simulink model "pid_test_model"  (R2018b)
settings: Solver=VariableStepAuto  StartTime=0.0  StopTime=2  RelTol=1e-3
libraries: nesl_utility x6, elec_lib x4, fl_lib x4, peGeneralControl x3, powerlib_meascontrol x2, simulink_extras x1
settings Model: Creator=macke  LastModifiedBy=macke

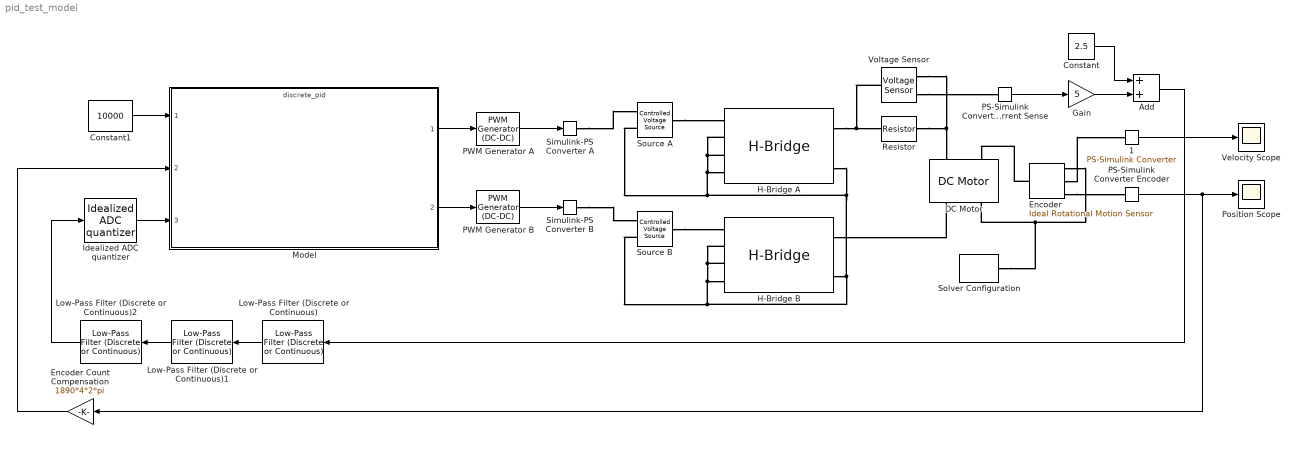
== system pid_test_model ==
  1 : nesl_utility/PS-Simulink Converter  PhysicalDomain=network_engine_domain  SubClassName=ps_output  LeftPortType=input  RightPortType=output  PseudoPeriodic=off  Frequencies=[]  Unit=1  AffineConversion=off
  Add : Sum
  Constant : Constant  Value=2.5
  Constant1 : Constant  Value=10000
  DC Motor : elec_lib/Actuators & Drivers/Rotational Actuators/DC Motor  parameterization=3  Ra=3.9 Ohm  La=12e-6 H  emf_or_torque=1  Kv=0.072e-3 V/rpm  Ki=6.876e-4 N*m/A  T_stall=0.24e-3 N*m  w_max=16.7 rpm  w_rated=12 rpm  P_rated=1.722 W  V_rated=12 V  J=0.01 g*cm^2  lam_param=2  lam=0 N*m/(rad/s)  i_noload=0.1 A  V_i_noload=12 V  speed0=0 rpm  alpha=3.93e-3 1/K  Tmeas=25 degC  thermal_mass=100 J/K  initial_temperature=25 degC
  Encoder : fl_lib/Mechanical/Mechanical Sensors/Ideal Rotational Motion Sensor  offset=0 rad
  Encoder Count Compensation : Gain  Gain=1890*4*2*pi
  Gain : Gain  Gain=5
  H-Bridge A : elec_lib/Actuators & Drivers/Drivers/H-Bridge  Venable=0.5 V  Vmax=1 V  Vreverse=0.5 V  Vbrake=0.5 V  Vm=12 V  pwm_or_av=1  discontinuous=0  freewheeling_mode=2  freewheeling_mode_disc=1  Ron=0.275 Ohm  Don=0.05 Ohm  Rload=10 Ohm  Lload=1e-5 H  F=10 kHz  thermal_mass=100 J/K  initial_temperature=298.15 K  Ron2=0.1 Ohm  Don2=0.05 Ohm  Tmeas=298.15 K  Tmeas2=398.15 K
      settings: SourceProductName=Simscape Electronics  SourceProductBaseCode=SN
  H-Bridge B : elec_lib/Actuators & Drivers/Drivers/H-Bridge  Venable=0.5 V  Vmax=1 V  Vreverse=0.5 V  Vbrake=0.5 V  Vm=12 V  pwm_or_av=1  discontinuous=0  freewheeling_mode=2  freewheeling_mode_disc=1  Ron=0.275 Ohm  Don=0.05 Ohm  Rload=10 Ohm  Lload=1e-5 H  F=10 kHz  thermal_mass=100 J/K  initial_temperature=298.15 K  Ron2=0.1 Ohm  Don2=0.05 Ohm  Tmeas=298.15 K  Tmeas2=398.15 K
      settings: SourceProductName=Simscape Electronics  SourceProductBaseCode=SN
  Idealized ADC quantizer : simulink_extras/Additional Discrete/Idealized ADC quantizer  NumberOfConverterBits=8  Vmin=0  Vmax=5  OutputDataType=uint8  OutputNegativeValues=off
      settings: SourceProductName=Simulink
  Low-Pass Filter (Discrete or Continuous) : peGeneralControl/Low-Pass Filter (Discrete or Continuous)  K=1  T=0.0002  B=inf  A=-inf  Ts=-1
  Low-Pass Filter (Discrete or Continuous)1 : peGeneralControl/Low-Pass Filter (Discrete or Continuous)  K=1  T=0.0002  B=inf  A=-inf  Ts=-1
  Low-Pass Filter (Discrete or Continuous)2 : peGeneralControl/Low-Pass Filter (Discrete or Continuous)  K=1  T=0.0002  B=inf  A=-inf  Ts=-1
  Model : ModelReference  ModelNameDialog=discrete_pid  SimulationMode=Normal  ModelReferenceVersion=1.21
  PS-Simulink Converter Current Sense : nesl_utility/PS-Simulink Converter  PhysicalDomain=network_engine_domain  SubClassName=ps_output  LeftPortType=input  RightPortType=output  PseudoPeriodic=off  Frequencies=[]  Unit=1  AffineConversion=off
  PS-Simulink Converter Encoder : nesl_utility/PS-Simulink Converter  PhysicalDomain=network_engine_domain  SubClassName=ps_output  LeftPortType=input  RightPortType=output  PseudoPeriodic=off  Frequencies=[]  Unit=1  AffineConversion=off
  PWM Generator A : powerlib_meascontrol/Pulse & Signal Generators/PWM Generator (DC-DC)  Fsw=31250*2  Ts=0
  PWM Generator B : powerlib_meascontrol/Pulse & Signal Generators/PWM Generator (DC-DC)  Fsw=31250*2  Ts=0
  Position Scope : Scope
  Resistor : elec_lib/Passive Devices/Resistor  R=0.5 Ohm  R_tol=5  enable_R_tol=0  tol_distribution=1  nSigma=4  enable_operating_limits=0  operating_limit_action=2  max_working_voltage=100 V  power_rating=1 W  enable_faults=0  fault_action=1  R_faulted=inf Ohm  enable_temporal_fault=0  t_fault=1 s  enable_behavioral_fault=0  max_permissible_current=1 A  t_fail_on_current=1 s  noise_mode=0  sample_time=1e-3 s  repeatability=1  auto_seed=989487740  user_seed=0  Tdevice=25 degC  alpha=3.93e-3 1/K  Tmeas=25 degC  thermal_mass=100 J/K  power_derating_T1=70 degC  power_derating_T2=155 degC  operating_temperature_range_vec=[-50, 150] degC  temperature_specify=off  temperature_priority=High  temperature=298.15 K  temperature_nominal_specify=off  temperature_nominal_unit=K  temperature_nominal_value=1
  Simulink-PS Converter A : nesl_utility/Simulink-PS Converter  PhysicalDomain=network_engine_domain  SubClassName=ps_input  LeftPortType=input  RightPortType=output  PseudoPeriodic=off  Frequencies=[]  NoiseDistribution=none  NoiseParameters=[]  Unit=V  AffineConversion=off  FilteringAndDerivatives=provide  SimscapeFilterOrder=1  InputFilterTimeConstant=0.001  UdotUserProvided=0
  Simulink-PS Converter B : nesl_utility/Simulink-PS Converter  PhysicalDomain=network_engine_domain  SubClassName=ps_input  LeftPortType=input  RightPortType=output  PseudoPeriodic=off  Frequencies=[]  NoiseDistribution=none  NoiseParameters=[]  Unit=V  AffineConversion=off  FilteringAndDerivatives=provide  SimscapeFilterOrder=1  InputFilterTimeConstant=0.001  UdotUserProvided=0
  Solver Configuration : nesl_utility/Solver Configuration  PhysicalDomain=network_engine_domain  SubClassName=solver  LeftPortType=input  RightPortType=generic  Tones=[]  Harmonics=[]  SimulateNoise=off  Profile=off  UseLocalSampling=off  EnableSwitchedLinearOptims=on  FrequencyDomain=off  UseCCode=off  RelTol=0.001  AbsTol=1e-06  MinStep=1e-09  ToWorkspace=off  RevertToSquareIcSolve=off  NumHomotopyIterations=100  PhasorMode=off  PhasorModeNumHarmonics=1  DoDC=off  ResidualTolerance=1e-09  UseLocalSolver=off  LocalSolverChoice=NE_BACKWARD_EULER_ADVANCER  LocalSolverSampleTime=0.001  DoFixedCost=off  MaxNonlinIter=3  MaxModeIter=2  LinearAlgebra=auto  EquationFormulation=NE_TIME_EF  DelaysMemoryBudget=1024  AutomaticFiltering=on  FilteringTimeConstant=0.001  PartitionStorageMethod=AS_NEEDED  PartitionMemoryBudget=1024
  Source A : fl_lib/Electrical/Electrical Sources/Controlled Voltage Source
  Source B : fl_lib/Electrical/Electrical Sources/Controlled Voltage Source
  Velocity Scope : Scope
  Voltage Sensor : fl_lib/Electrical/Electrical Sensors/Voltage Sensor
  wires:
  Model/1 -> PWM Generator A/1
  Model/2 -> PWM Generator B/1
  PWM Generator A/1 -> Simulink-PS Converter A/1
  PWM Generator B/1 -> Simulink-PS Converter B/1
  PS-Simulink Converter Current Sense/1 -> Gain/1
  Constant/1 -> Add/1
  Gain/1 -> Add/2
  Low-Pass Filter (Discrete or Continuous)/1 -> Low-Pass Filter (Discrete or Continuous)1/1
  Low-Pass Filter (Discrete or Continuous)1/1 -> Low-Pass Filter (Discrete or Continuous)2/1
  Add/1 -> Low-Pass Filter (Discrete or Continuous)/1
  Idealized ADC quantizer/1 -> Model/3
  Low-Pass Filter (Discrete or Continuous)2/1 -> Idealized ADC quantizer/1
  Constant1/1 -> Model/1
  1/1 -> Velocity Scope/1
  PS-Simulink Converter Encoder/1 -> Encoder Count Compensation/1, Position Scope/1
  Encoder Count Compensation/1 -> Model/2
  connections:
  Source A/LConn1 -- H-Bridge A/LConn1
  Simulink-PS Converter A/RConn1 -- Source A/RConn1
  Source B/RConn2 -- H-Bridge B/RConn2 -- H-Bridge A/RConn2 -- H-Bridge A/LConn3 -- H-Bridge A/LConn2 -- H-Bridge A/LConn4 -- Source A/RConn2 -- H-Bridge B/LConn3 -- H-Bridge B/LConn2 -- H-Bridge B/LConn4
  Simulink-PS Converter B/RConn1 -- Source B/RConn1
  Source B/LConn1 -- H-Bridge B/LConn1
  H-Bridge B/RConn1 -- DC Motor/RConn1
  H-Bridge A/RConn1 -- Voltage Sensor/LConn1 -- Resistor/LConn1
  Resistor/RConn1 -- Voltage Sensor/RConn2 -- DC Motor/LConn1
  Voltage Sensor/RConn1 -- PS-Simulink Converter Current Sense/LConn1
  Encoder/LConn1 -- DC Motor/LConn2
  Encoder/RConn1 -- Solver Configuration/RConn1 -- DC Motor/RConn2
  Encoder/RConn3 -- PS-Simulink Converter Encoder/LConn1
  Encoder/RConn2 -- 1/LConn1
